simulink model "momentum_unload_test"  (R2016b)
settings: Solver=VariableStepAuto  StartTime=0.0  StopTime=1500  MinStep=0.000001  RelTol=1e-3
values from neighbouring files (symbols this model uses):
  fsw_params = init_fsw_params()    [momentum_unload_test_init.m]
undefined symbols (not defined in the file or in its folder): DiscIntNeverNeededParam
libraries: aerolibutil x3, dynamics_lib x1, environment_lib x1, momentum_dump_lib_test x1, RW_assembly_simple_lib x1, actuators_lib x1
settings Model: Creator=taylorreynolds  LastModifiedBy=evich

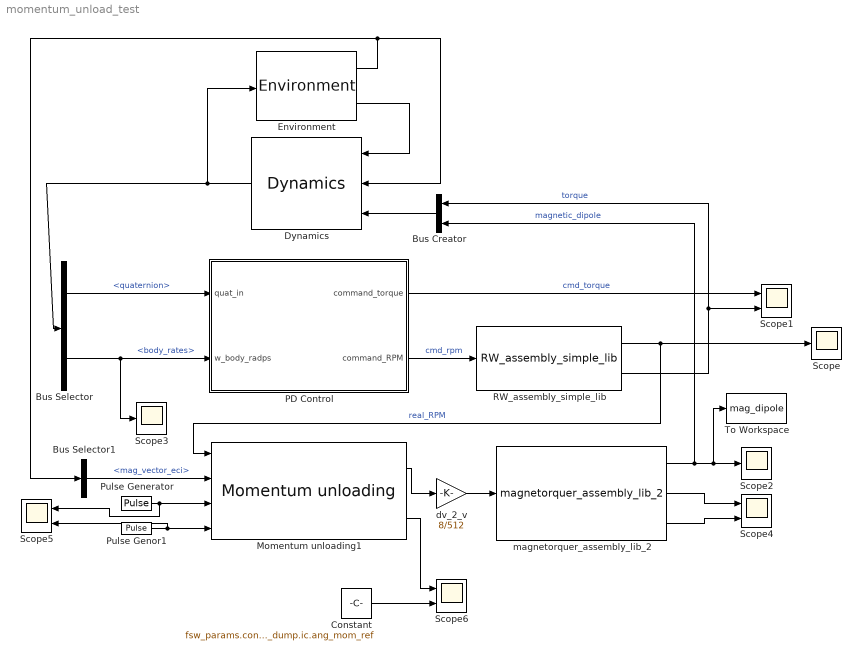
== system momentum_unload_test ==
  Bus Creator : BusCreator  Inputs=2
  Bus Selector : BusSelector  OutputSignals=quaternion,body_rates
  Bus Selector1 : BusSelector  OutputSignals=mag_vector_eci
  Constant : Constant  Value=fsw_params.control.p_dump.ic.ang_mom_ref
  Dynamics : dynamics_lib/Dynamics
  Environment : environment_lib/Environment
  Momentum unloading1 : momentum_dump_lib_test/Momentum unloading
  PD Control : Subsystem  AncestorBlock=pd_control_lib/PD Control
  Pulse Generator : DiscretePulseGenerator  PulseType=Time based  Period=fsw_params.actuators.ppt.sync_pulse  PulseWidth=fsw_params.actuators.ppt.t_charge_pct
  Pulse Genor1 : DiscretePulseGenerator  PulseType=Time based  Period=10  PulseWidth=sim_params.sensors.magnetometer.valid_pct
  RW_assembly_simple_lib : RW_assembly_simple_lib/RW_assembly_simple_lib  natural_frequency=100  damping_ratio=1  max_rate=100
  Scope : Scope
  Scope{1,4..6} (4 alike) : Scope  NumInputPorts=2
  Scope2 : Scope
  Scope3 : Scope
  To Workspace : ToWorkspace  VariableName=mag_dipole  SaveFormat=Timeseries  SampleTime=-1
  dv_2_v : Gain  Gain=8/512
  magnetorquer_assembly_lib_2 : actuators_lib/Actuators/magnetorquer_assembly_lib_2
  wires:
  Environment/2 -> Dynamics/1
  Environment/1 -> Dynamics/2, Bus Selector1/1
  Dynamics/1 -> Environment/1, Bus Selector/1
  Bus Selector/2 -> Scope3/1, PD Control/2(w_body_radps)  "<body_rates>"
  Bus Selector/1 -> PD Control/1(quat_in)  "<quaternion>"
  Bus Creator/1 -> Dynamics/3
  magnetorquer_assembly_lib_2/1 -> Scope2/1, To Workspace/1, Bus Creator/2  "magnetic_dipole"
  PD Control/2(command_RPM) -> RW_assembly_simple_lib/1  "cmd_rpm"
  RW_assembly_simple_lib/2 -> Bus Creator/1, Scope1/2  "torque"
  PD Control/1(command_torque) -> Scope1/1  "cmd_torque"
  RW_assembly_simple_lib/1 -> Momentum unloading1/1, Scope/1  "real_RPM"
  Momentum unloading1/1 -> dv_2_v/1
  magnetorquer_assembly_lib_2/2 -> Scope4/1
  magnetorquer_assembly_lib_2/3 -> Scope4/2
  Bus Selector1/1 -> Momentum unloading1/2  "<mag_vector_eci>"
  Pulse Generator/1 -> Momentum unloading1/3, Scope5/1
  Pulse Genor1/1 -> Momentum unloading1/4, Scope5/2
  dv_2_v/1 -> magnetorquer_assembly_lib_2/1
  Momentum unloading1/2 -> Scope6/1
  Constant/1 -> Scope6/2

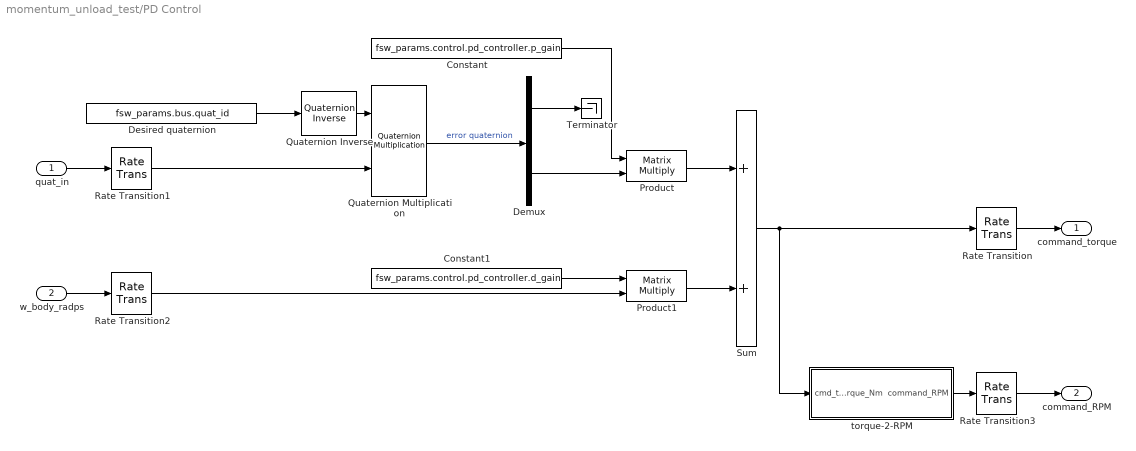
== system momentum_unload_test/PD Control ==
  quat_in : Inport
  w_body_radps : Inport  Port=2
  Constant : Constant  Value=fsw_params.control.pd_controller.p_gain
  Constant1 : Constant  Value=fsw_params.control.pd_controller.d_gain
  Demux : Demux  Outputs=[1 3]
  Desired quaternion : Constant  Value=fsw_params.bus.quat_id
  Product : Product  Multiplication=Matrix(*)
  Product1 : Product  Multiplication=Matrix(*)
  Quaternion Inverse : aerolibutil/Quaternion Inverse
  Quaternion Multiplication : aerolibutil/Quaternion Multiplication
  Rate Transition : RateTransition  X0=fsw_params.control.pd_controller.ic.rt_command_torque
  Rate Transition1 : RateTransition  X0=fsw_params.control.pd_controller.ic.rt_quat_in  OutPortSampleTime=fsw_params.control.pd_controller.sample_time_s
  Rate Transition2 : RateTransition  X0=fsw_params.control.pd_controller.ic.rt_w_body_radps  OutPortSampleTime=fsw_params.control.pd_controller.sample_time_s
  Rate Transition3 : RateTransition  X0=fsw_params.control.pd_controller.ic.rt_command_RPM
  Sum : Sum
  Terminator : Terminator
  torque-2-RPM : Subsystem
  command_torque : Outport
  command_RPM : Outport  Port=2
  wires:
  torque-2-RPM/1(command_RPM) -> Rate Transition3/1
  Rate Transition3/1 -> command_RPM/1
  Rate Transition2/1 -> Product1/2
  Rate Transition1/1 -> Quaternion Multiplication/2
  Rate Transition/1 -> command_torque/1
  Sum/1 -> Rate Transition/1, torque-2-RPM/1(cmd_torque_Nm)
  Product1/1 -> Sum/2
  Product/1 -> Sum/1
  Demux/2 -> Product/2
  w_body_radps/1 -> Rate Transition2/1
  Demux/1 -> Terminator/1
  Quaternion Multiplication/1 -> Demux/1  "error quaternion"
  quat_in/1 -> Rate Transition1/1
  Quaternion Inverse/1 -> Quaternion Multiplication/1
  Desired quaternion/1 -> Quaternion Inverse/1
  Constant/1 -> Product/1
  Constant1/1 -> Product1/1

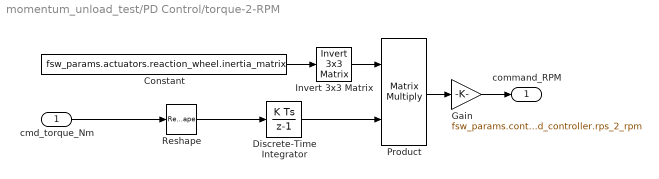
== system momentum_unload_test/PD Control/torque-2-RPM ==
  cmd_torque_Nm : Inport
  Constant : Constant  Value=fsw_params.actuators.reaction_wheel.inertia_matrix
  Discrete-Time Integrator : DiscreteIntegrator  InitialCondition=fsw_params.control.pd_controller.ic.torque  InitialConditionSetting=State (most efficient)  SampleTime=-1  ICPrevOutput=DiscIntNeverNeededParam  ICPrevScaledInput=DiscIntNeverNeededParam
  Gain : Gain  Gain=fsw_params.control.pd_controller.rps_2_rpm
  Invert 3x3 Matrix : aerolibutil/Invert  3x3 Matrix
  Product : Product  Multiplication=Matrix(*)
  Reshape : Reshape  OutputDimensionality=Column vector (2-D)  OutputDimensions=[3,1]
  command_RPM : Outport
  wires:
  Discrete-Time Integrator/1 -> Product/2
  Reshape/1 -> Discrete-Time Integrator/1
  Gain/1 -> command_RPM/1
  Product/1 -> Gain/1
  Invert 3x3 Matrix/1 -> Product/1
  Constant/1 -> Invert 3x3 Matrix/1
  cmd_torque_Nm/1 -> Reshape/1
